simulink model "CSE_STEPRESPONSE_BLOCKDIAGRAM_NO1_MAGSINO"  (R2019a)
settings: Solver=VariableStepAuto  StartTime=0.0  StopTime=20  RelTol=1e-3
values from neighbouring files (symbols this model uses):
  G_den1 = [b c d]    [CSE_STEPRESPONSE_CODE_NO1_MAGSINO.m]    (also in CSE_STEPRESPONSE_CODE_NO1_NO2_MAGSINO.m)
  G_num1 = [a]    [CSE_STEPRESPONSE_CODE_NO1_MAGSINO.m]    (also in CSE_STEPRESPONSE_CODE_NO1_NO2_MAGSINO.m)
settings Model: Creator=User  LastModifiedBy=User

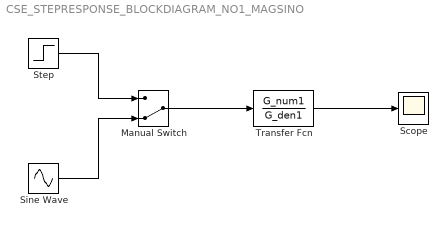
== system CSE_STEPRESPONSE_BLOCKDIAGRAM_NO1_MAGSINO ==
  Manual Switch : ManualSwitch  CurrentSetting=0
  Scope : Scope
  Sine Wave : Sin  SampleTime=0
  Step : Step  Time=0  SampleTime=0
  Transfer Fcn : TransferFcn  Numerator=G_num1  Denominator=G_den1
  wires:
  Step/1 -> Manual Switch/1
  Sine Wave/1 -> Manual Switch/2
  Manual Switch/1 -> Transfer Fcn/1
  Transfer Fcn/1 -> Scope/1
